simulink model "Nonlinear_Airframe"  (R2022a)
settings: Solver=FixedStepAuto  StartTime=0.0  StopTime=100.0  RelTol=1e-3
PreLoadFcn:
  | initScaleModel;
InitFcn:
  | initScaleModel
model workspace (MAT data in the model file):
  op_trim1 : opcond.OperatingReport (value not decoded)
undefined symbols (not defined in the file or in its folder): CG, coeffMatrix, CP, CT, mass
libraries: aerolibanim x2, aerolibasang x2, aerolibadyn x1, aerolibatmos2 x1, shared6dof x1
settings Model: Creator=natha  LastModifiedBy=natha
settings DataIOCC: ExternalInput=getinputstruct(op_trim1)  InitialState=getstatestruct(op_trim1)  LoadExternalInput=on  LoadInitialState=on  SaveOutput=off  SaveTime=off
settings OptimizationCC: EnhancedBackFolding=on  PassReuseOutputArgsAs=Individual arguments  ZeroExternalMemoryAtStartup=off  ZeroInternalMemoryAtStartup=off  MaxStackSize=64  OptimizeBlockOrder=speed  DifferentSizesBufferReuse=on  EfficientTunableParamExpr=on
settings DebuggingCC: ParameterTunabilityLossMsg=error
settings HardwareCC: UseEmbeddedCoderFeatures=off
settings SFSimCC: MATLABDynamicMemAlloc=off
settings RTWCC: SystemTargetFile=ert.tlc  HardwareBoard=Robot Operating System 2 (ROS 2)  TLCOptions="-aInlineSetEventsForThisBaseRateFcn=TLC_FALSE -aSuppressMultiTaskScheduler=TLC_FALSE  -aRateBasedStepFcn=0"  TemplateMakefile=ert_default_tmf  Toolchain=Colcon Tools  TargetLang=C++
settings CodeAppCC: ForceParamTrailComments=on  IgnoreCustomStorageClasses=off  OperatorAnnotations=on  SimulinkDataObjDesc=on  SFDataObjDesc=on  InsertBlockDesc=on
settings ERTTargetCC: CodeInterfacePackaging=C++ class  SupportNonInlinedSFcns=on  RootIOFormat=Structure reference

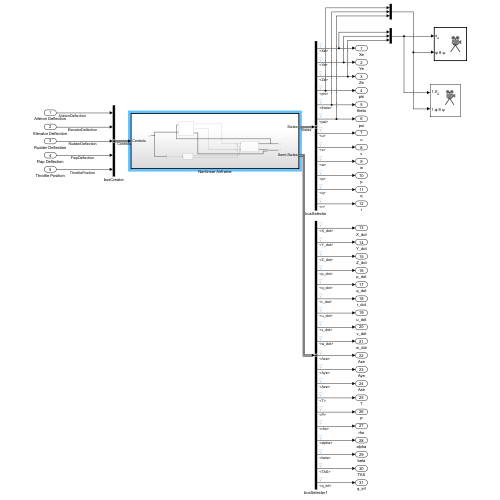
[thumbnail: Simulink's stored preview of the top-level diagram]
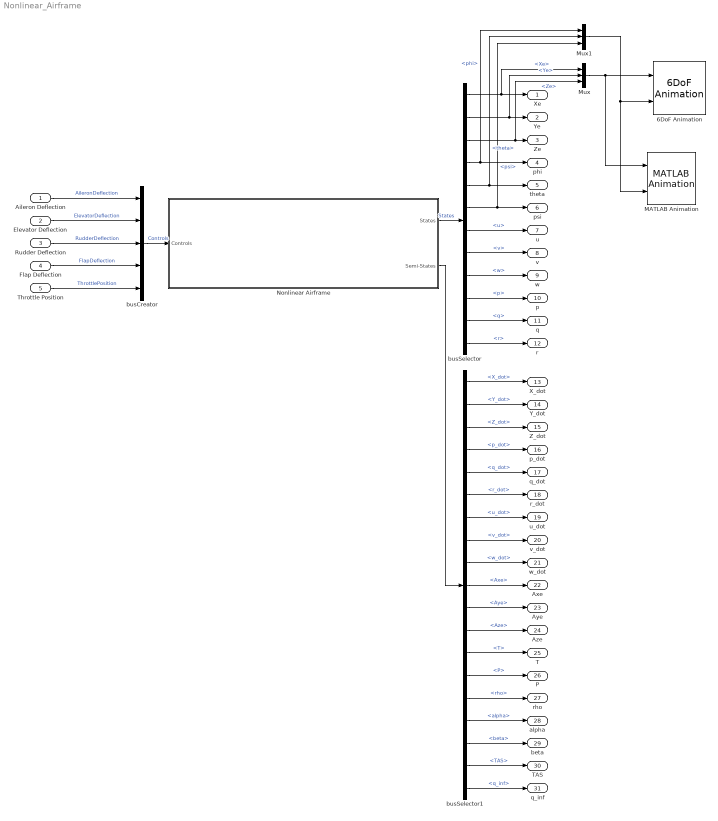
== system Nonlinear_Airframe ==
  Aileron Deflection : Inport
  Elevator Deflection : Inport  Port=2
  Rudder Deflection : Inport  Port=3
  Flap Deflection : Inport  Port=4
  Throttle Position : Inport  Port=5
  6DoF Animation : aerolibanim/6DoF Animation  u1=[0 4000 -2000 2000 -5000 -3000]  u2=0.1  u3=1.0  u4=[4000 0 -5000]  u5=Fixed position  u6=[2000 500 -3150]  u7=10  u8=on
  MATLAB Animation : aerolibanim/MATLAB Animation  Tag=Matlab Animation 6 DOF  Vehicles=1  Geometries='astredwedge.mat'  BoundingBoxCoordinates=[-50,50,-50,50,-50,50]  CameraOffset=[-150,-50,0]  CameraViewAngle=3  SampleTime=0.2  FigurePosition=[403,303,275,214]
      settings: SourceProductBaseCode=AE
  Mux : Mux  Inputs=3
  Mux1 : Mux  Inputs=3
  Nonlinear Airframe : Subsystem  TreatAsAtomicUnit=on
  busCreator : BusCreator  Inputs=5
  busSelector : BusSelector  OutputSignals=Xe,Ye,Ze,phi,theta,psi,u,v,w,p,q,r
  busSelector1 : BusSelector  OutputSignals=Semi-States.X_dot,Semi-States.Y_dot,Semi-States.Z_dot,Semi-States.p_dot,Semi-States.q_dot,Semi-States.r_dot,Semi-States.u_dot,Semi-States.v_dot,Semi-States.w_dot,Semi-States.Axe,Semi-States.Aye,Semi-States.Aze,Aero Semi-States.T,Aero Semi-States.P,Aero Semi-States.rho,Aero Semi-States.alpha,Aero Semi-States.beta,Aero Semi-States.TAS,Aero Semi-States.q_inf
  Xe : Outport
  Ye : Outport  Port=2
  Ze : Outport  Port=3
  phi : Outport  Port=4
  theta : Outport  Port=5
  psi : Outport  Port=6
  u : Outport  Port=7
  v : Outport  Port=8
  w : Outport  Port=9
  p : Outport  Port=10
  q : Outport  Port=11
  r : Outport  Port=12
  X_dot : Outport  Port=13
  Y_dot : Outport  Port=14
  Z_dot : Outport  Port=15
  p_dot : Outport  Port=16
  q_dot : Outport  Port=17
  r_dot : Outport  Port=18
  u_dot : Outport  Port=19
  v_dot : Outport  Port=20
  w_dot : Outport  Port=21
  Axe : Outport  Port=22
  Aye : Outport  Port=23
  Aze : Outport  Port=24
  T : Outport  Port=25
  P : Outport  Port=26
  rho : Outport  Port=27
  alpha : Outport  Port=28
  beta : Outport  Port=29
  TAS : Outport  Port=30
  q_inf : Outport  Port=31
  wires:
  busSelector1/17 -> beta/1  "<beta>"
  busSelector1/19 -> q_inf/1  "<q_inf>"
  busSelector1/18 -> TAS/1  "<TAS>"
  Nonlinear Airframe/2(Semi-States) -> busSelector1/1
  busSelector1/16 -> alpha/1  "<alpha>"
  busSelector1/15 -> rho/1  "<rho>"
  busSelector1/13 -> T/1  "<T>"
  busSelector1/12 -> Aze/1  "<Aze>"
  Nonlinear Airframe/1(States) -> busSelector/1  "States"
  busSelector1/14 -> P/1  "<P>"
  busSelector1/11 -> Aye/1  "<Aye>"
  busSelector1/9 -> w_dot/1  "<w_dot>"
  busSelector1/10 -> Axe/1  "<Axe>"
  busSelector1/8 -> v_dot/1  "<v_dot>"
  busSelector1/6 -> r_dot/1  "<r_dot>"
  busSelector1/7 -> u_dot/1  "<u_dot>"
  busSelector1/5 -> q_dot/1  "<q_dot>"
  busSelector1/4 -> p_dot/1  "<p_dot>"
  busSelector1/3 -> Z_dot/1  "<Z_dot>"
  busSelector1/1 -> X_dot/1  "<X_dot>"
  busSelector1/2 -> Y_dot/1  "<Y_dot>"
  busSelector/12 -> r/1  "<r>"
  busSelector/9 -> w/1  "<w>"
  busSelector/11 -> q/1  "<q>"
  busSelector/10 -> p/1  "<p>"
  busSelector/5 -> Mux1/2, theta/1  "<theta>"
  busSelector/7 -> u/1  "<u>"
  busSelector/8 -> v/1  "<v>"
  busSelector/6 -> Mux1/3, psi/1  "<psi>"
  busSelector/2 -> Ye/1, Mux/2  "<Ye>"
  busSelector/3 -> Ze/1, Mux/3  "<Ze>"
  busSelector/4 -> Mux1/1, phi/1  "<phi>"
  busSelector/1 -> Xe/1, Mux/1  "<Xe>"
  Throttle Position/1 -> busCreator/5  "ThrottlePosition"
  Flap Deflection/1 -> busCreator/4  "FlapDeflection"
  Rudder Deflection/1 -> busCreator/3  "RudderDeflection"
  Elevator Deflection/1 -> busCreator/2  "ElevatorDeflection"
  Aileron Deflection/1 -> busCreator/1  "AileronDeflection"
  busCreator/1 -> Nonlinear Airframe/1(Controls)  "Controls"
  Mux/1 -> MATLAB Animation/1, 6DoF Animation/1
  Mux1/1 -> MATLAB Animation/2, 6DoF Animation/2

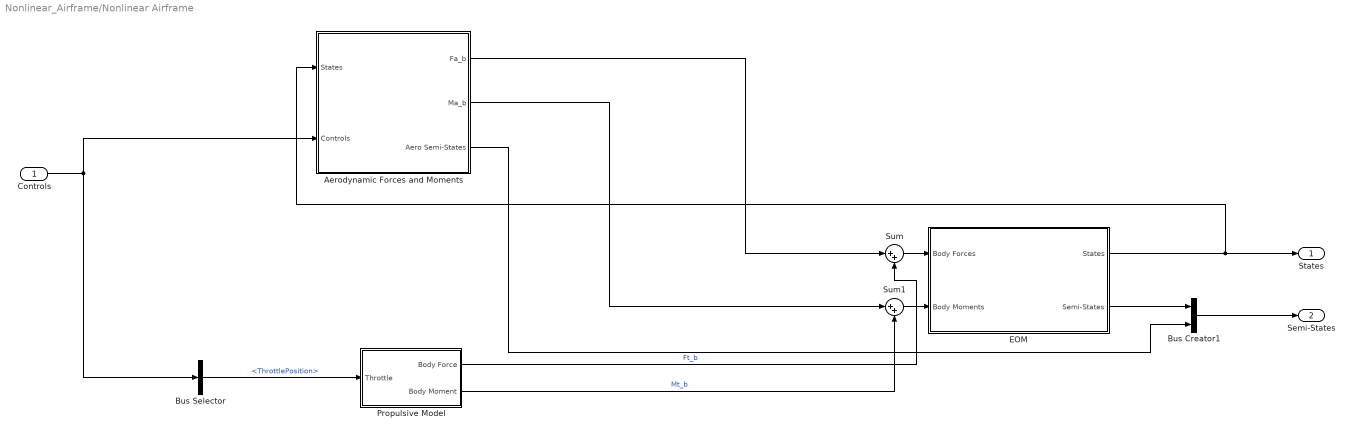
== system Nonlinear_Airframe/Nonlinear Airframe ==
  Controls : Inport
  Aerodynamic Forces and Moments : Subsystem
  Bus Creator1 : BusCreator  Inputs=2
  Bus Selector : BusSelector  OutputSignals=ThrottlePosition
  EOM : Subsystem
  Propulsive Model : Subsystem
  Sum : Sum  Inputs=|++
  Sum1 : Sum  Inputs=|++
  States : Outport
  Semi-States : Outport  Port=2
  wires:
  Aerodynamic Forces and Moments/3(Aero Semi-States) -> Bus Creator1/2
  Bus Selector/1 -> Propulsive Model/1(Throttle)  "<ThrottlePosition>"
  Bus Creator1/1 -> Semi-States/1
  Controls/1 -> Aerodynamic Forces and Moments/2(Controls), Bus Selector/1
  Aerodynamic Forces and Moments/2(Ma_b) -> Sum1/1
  Aerodynamic Forces and Moments/1(Fa_b) -> Sum/1
  Sum1/1 -> EOM/2(Body Moments)
  Propulsive Model/2(Body Moment) -> Sum1/2  "Mt_b"
  Propulsive Model/1(Body Force) -> Sum/2  "Ft_b"
  Sum/1 -> EOM/1(Body Forces)
  EOM/2(Semi-States) -> Bus Creator1/1
  EOM/1(States) -> States/1, Aerodynamic Forces and Moments/1(States)

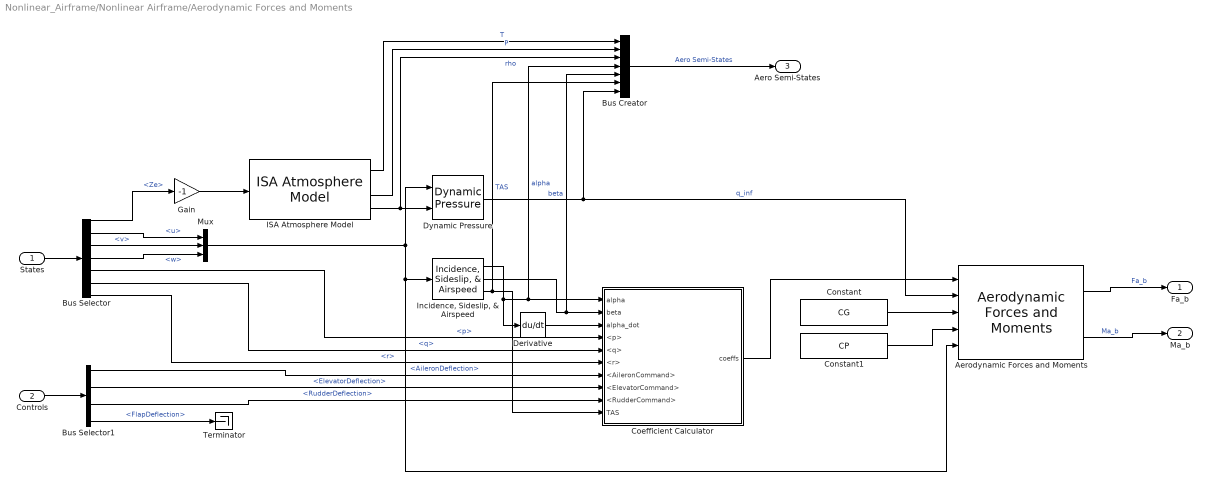
== system Nonlinear_Airframe/Nonlinear Airframe/Aerodynamic Forces and Moments ==
  States : Inport
  Controls : Inport  Port=2
  "Aerodynamic Forces and Moments " : aerolibadyn/Aerodynamic Forces and Moments   inputAxes=Stability  outputForceAxes=Body  outputMomentAxes=Body  S=0.342  b=1.667  cbar=0.205
  Bus Creator : BusCreator  Inputs=7
  Bus Selector : BusSelector  OutputSignals=Ze,u,v,w,p,q,r
  Bus Selector1 : BusSelector  OutputSignals=AileronDeflection,ElevatorDeflection,RudderDeflection,FlapDeflection
  Coefficient Calculator : Subsystem
  Constant : Constant  Value=CG
  Constant1 : Constant  Value=CP
  Derivative : Derivative
  Dynamic Pressure : aerolibasang/Dynamic Pressure
  Gain : Gain  Gain=-1
  ISA Atmosphere Model : aerolibatmos2/ISA Atmosphere Model  custom=off  g=9.80665  gamma=1.4  R=287.0531  L=0.0065  h_trop=11000  h_strat=20000  rho0=1.225  P0=101325  T0=288.15  h0=0
  "Incidence, Sideslip, & Airspeed" : aerolibasang/Incidence, Sideslip, & Airspeed
  Mux : Mux  Inputs=3
  Terminator : Terminator
  Fa_b : Outport
  Ma_b : Outport  Port=2
  Aero Semi-States : Outport  Port=3
  wires:
  ISA Atmosphere Model/3 -> Bus Creator/2  "P"
  ISA Atmosphere Model/1 -> Bus Creator/1  "T"
  Bus Creator/1 -> Aero Semi-States/1  "Aero Semi-States"
  Coefficient Calculator/1(coeffs) -> "Aerodynamic Forces and Moments "/1
  "Incidence, Sideslip, & Airspeed"/3 -> Coefficient Calculator/10(TAS), Bus Creator/6  "TAS"
  Bus Selector1/3 -> Coefficient Calculator/9(<RudderCommand>)  "<RudderDeflection>"
  Bus Selector1/2 -> Coefficient Calculator/8(<ElevatorCommand>)  "<ElevatorDeflection>"
  Bus Selector1/1 -> Coefficient Calculator/7(<AileronCommand>)  "<AileronDeflection>"
  Bus Selector/7 -> Coefficient Calculator/6(<r>)  "<r>"
  Bus Selector/6 -> Coefficient Calculator/5(<q>)  "<q>"
  Bus Selector/5 -> Coefficient Calculator/4(<p>)  "<p>"
  "Incidence, Sideslip, & Airspeed"/2 -> Coefficient Calculator/2(beta), Bus Creator/5  "beta"
  Derivative/1 -> Coefficient Calculator/3(alpha_dot)
  Bus Selector1/4 -> Terminator/1  "<FlapDeflection>"
  Controls/1 -> Bus Selector1/1
  "Incidence, Sideslip, & Airspeed"/1 -> Derivative/1, Coefficient Calculator/1(alpha), Bus Creator/4  "alpha"
  "Aerodynamic Forces and Moments "/1 -> Fa_b/1  "Fa_b"
  "Aerodynamic Forces and Moments "/2 -> Ma_b/1  "Ma_b"
  Mux/1 -> "Incidence, Sideslip, & Airspeed"/1, "Aerodynamic Forces and Moments "/5, Dynamic Pressure/1
  Gain/1 -> ISA Atmosphere Model/1
  Constant1/1 -> "Aerodynamic Forces and Moments "/4
  Constant/1 -> "Aerodynamic Forces and Moments "/3
  Bus Selector/4 -> Mux/3  "<w>"
  Bus Selector/2 -> Mux/1  "<u>"
  Bus Selector/1 -> Gain/1  "<Ze>"
  States/1 -> Bus Selector/1
  Bus Selector/3 -> Mux/2  "<v>"
  ISA Atmosphere Model/4 -> Dynamic Pressure/2, Bus Creator/3  "rho"
  Dynamic Pressure/1 -> "Aerodynamic Forces and Moments "/2, Bus Creator/7  "q_inf"

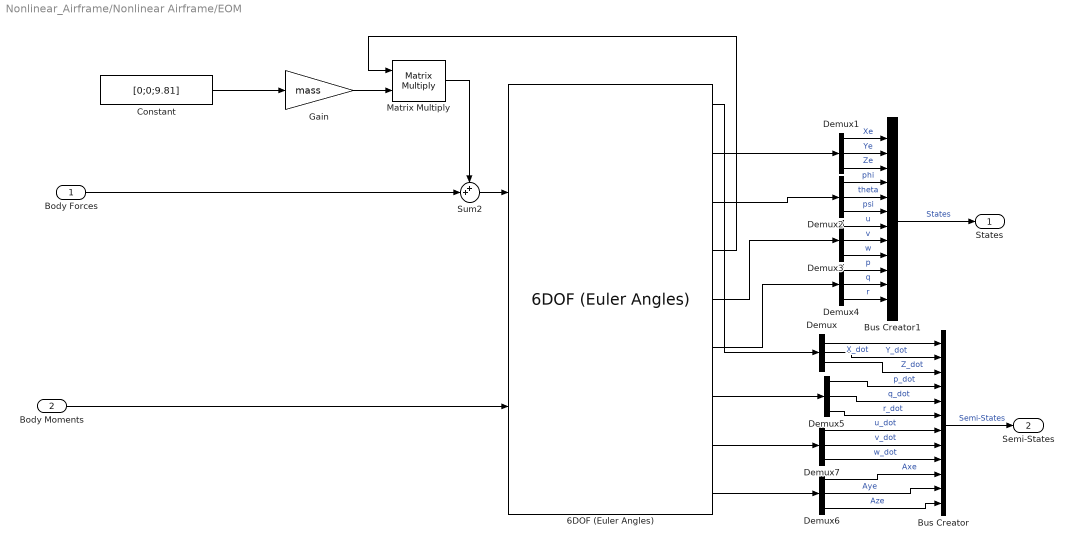
== system Nonlinear_Airframe/Nonlinear Airframe/EOM ==
  Body Forces : Inport
  Body Moments : Inport  Port=2
  6DOF (Euler Angles) : shared6dof/6DOF (Euler Angles)  units=Metric (MKS)  mtype=Fixed  rep=Euler Angles  xme_0=[0 0 -91.44]  Vm_0=[10 0 0]  eul_0=[0 0 0]  pm_0=[0 0 0]  mass_0=mass  mass_e=0.5  mass_f=2.0  inertia=inertia  inertia_e=eye(3)  inertia_f=2*eye(3)  k_quat=1.0  vre_flag=on  abi_flag=on  aMode=0  xme_statename={'Xe', 'Ye', 'Ze'}  Vm_statename={'u', 'v', 'w'}  eul_statename={'phi', 'theta', 'psi'}  quat_statename={'qr', 'qi', 'qj','qk'}  pm_statename={'p', 'q', 'r'}  mass_statename=''
      settings: SourceProductBaseCode=AE,PW,DR,MT,VE
  Bus Creator1 : BusCreator  Inputs=12
  Bus Creator : BusCreator  Inputs=12
  Constant : Constant  Value=[0;0;9.81]  VectorParams1D=off
  Demux{,1..7} (8 alike) : Demux  Outputs=3
  Gain : Gain  Gain=mass
  Matrix Multiply : Product  Multiplication=Matrix(*)
  Sum2 : Sum  Inputs=++|  InputSameDT=on  SaturateOnIntegerOverflow=on  OutDataTypeStr=Inherit: Same as first input
  States : Outport
  Semi-States : Outport  Port=2
  wires:
  Demux/3 -> Bus Creator/3  "Z_dot"
  Demux/2 -> Bus Creator/2  "Y_dot"
  Demux/1 -> Bus Creator/1  "X_dot"
  Demux7/3 -> Bus Creator/9  "w_dot"
  Demux7/2 -> Bus Creator/8  "v_dot"
  Demux7/1 -> Bus Creator/7  "u_dot"
  6DOF (Euler Angles)/8 -> Demux7/1
  Bus Creator1/1 -> States/1  "States"
  Body Forces/1 -> Sum2/2
  6DOF (Euler Angles)/6 -> Demux4/1
  Matrix Multiply/1 -> Sum2/1
  Demux4/3 -> Bus Creator1/12  "r"
  Demux3/3 -> Bus Creator1/9  "w"
  Demux3/2 -> Bus Creator1/8  "v"
  Demux3/1 -> Bus Creator1/7  "u"
  Body Moments/1 -> 6DOF (Euler Angles)/2
  Demux2/2 -> Bus Creator1/5  "theta"
  Bus Creator/1 -> Semi-States/1  "Semi-States"
  Demux2/3 -> Bus Creator1/6  "psi"
  Demux2/1 -> Bus Creator1/4  "phi"
  Demux1/3 -> Bus Creator1/3  "Ze"
  Demux1/2 -> Bus Creator1/2  "Ye"
  Demux4/1 -> Bus Creator1/10  "p"
  6DOF (Euler Angles)/7 -> Demux5/1
  Demux4/2 -> Bus Creator1/11  "q"
  Demux6/3 -> Bus Creator/12  "Aze"
  Demux6/2 -> Bus Creator/11  "Aye"
  6DOF (Euler Angles)/5 -> Demux3/1
  6DOF (Euler Angles)/3 -> Demux2/1
  Demux6/1 -> Bus Creator/10  "Axe"
  Demux5/1 -> Bus Creator/4  "p_dot"
  Demux5/2 -> Bus Creator/5  "q_dot"
  Sum2/1 -> 6DOF (Euler Angles)/1
  Demux1/1 -> Bus Creator1/1  "Xe"
  6DOF (Euler Angles)/9 -> Demux6/1
  Constant/1 -> Gain/1
  6DOF (Euler Angles)/4 -> Matrix Multiply/1
  6DOF (Euler Angles)/1 -> Demux/1
  Demux5/3 -> Bus Creator/6  "r_dot"
  Gain/1 -> Matrix Multiply/2
  6DOF (Euler Angles)/2 -> Demux1/1

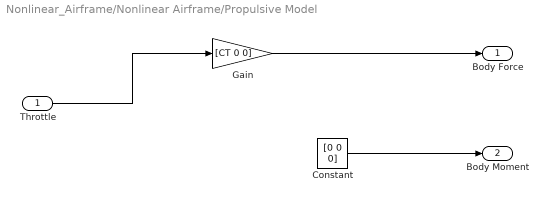
== system Nonlinear_Airframe/Nonlinear Airframe/Propulsive Model ==
  Throttle : Inport
  Constant : Constant  Value=[0 0 0]
  Gain : Gain  Gain=[CT 0 0]
  Body Force : Outport
  Body Moment : Outport  Port=2
  wires:
  Throttle/1 -> Gain/1
  Gain/1 -> Body Force/1
  Constant/1 -> Body Moment/1

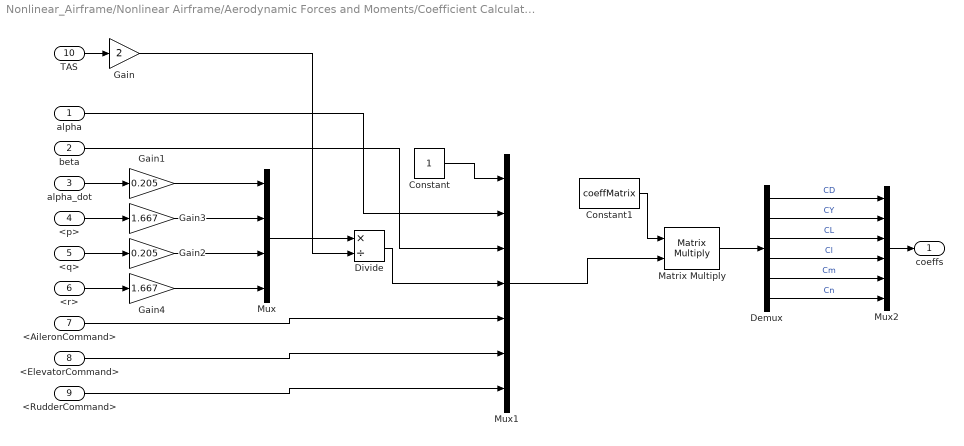
== system Nonlinear_Airframe/Nonlinear Airframe/Aerodynamic Forces and Moments/Coefficient Calculator ==
  alpha : Inport
  beta : Inport  Port=2
  alpha_dot : Inport  Port=3
  <p> : Inport  Port=4
  <q> : Inport  Port=5
  <r> : Inport  Port=6
  <AileronCommand> : Inport  Port=7
  <ElevatorCommand> : Inport  Port=8
  <RudderCommand> : Inport  Port=9
  TAS : Inport  Port=10
  Constant : Constant
  Constant1 : Constant  Value=coeffMatrix
  Demux : Demux  Outputs=6
  Divide : Product  Inputs=*/
  Gain : Gain  Gain=2
  Gain1 : Gain  Gain=0.205
  Gain2 : Gain  Gain=0.205
  Gain3 : Gain  Gain=1.667
  Gain4 : Gain  Gain=1.667
  Matrix Multiply : Product  Multiplication=Matrix(*)
  Mux : Mux
  Mux1 : Mux  Inputs=7
  Mux2 : Mux  Inputs=6
  coeffs : Outport
  wires:
  Constant1/1 -> Matrix Multiply/1
  Mux1/1 -> Matrix Multiply/2
  <RudderCommand>/1 -> Mux1/7
  <ElevatorCommand>/1 -> Mux1/6
  <AileronCommand>/1 -> Mux1/5
  Divide/1 -> Mux1/4
  beta/1 -> Mux1/3
  alpha/1 -> Mux1/2
  Constant/1 -> Mux1/1
  Gain/1 -> Divide/2
  Mux/1 -> Divide/1
  Gain4/1 -> Mux/4
  Gain3/1 -> Mux/2
  Gain2/1 -> Mux/3
  Gain1/1 -> Mux/1
  <r>/1 -> Gain4/1
  <p>/1 -> Gain3/1
  <q>/1 -> Gain2/1
  alpha_dot/1 -> Gain1/1
  TAS/1 -> Gain/1
  Matrix Multiply/1 -> Demux/1
  Mux2/1 -> coeffs/1
  Demux/1 -> Mux2/1  "CD"
  Demux/2 -> Mux2/2  "CY"
  Demux/3 -> Mux2/3  "CL"
  Demux/4 -> Mux2/4  "Cl"
  Demux/5 -> Mux2/5  "Cm"
  Demux/6 -> Mux2/6  "Cn"
